simulink model "Main1"  (R2017b)
settings: Solver=ode15s  StartTime=0.0  StopTime=t_end  FixedStep=.0001  MaxStep=st  RelTol=1e-3  EnableMultiTasking=on
values from neighbouring files (symbols this model uses):
  A = eye(16,16)    [full_input_list.m]
  B = zeros(16,1)    [full_input_list.m]
  C = blkdiag(eye(3,3),zeros(3,3),eye(10,10))    [full_input_list.m]
  deltaT = 0.00001    (= 1e-05)    [full_input_list.m]
  H = C    [full_input_list.m]
  I_UD = [0.032808359, 0.000617048, 0.000049185;      0.000617048, 0.032531573, 0.000060042;      0.000049185, 0.000060042, 0.007799591]    [full_input_list.m]
  kd = 0.5    [full_input_list.m]    (also in initACS.m = 0.01)
  kd_UD_detumble = 6e-3    (= 0.006)    [full_input_list.m]
  kd_UD_slew = epsilon_UD_slew*.3    (= 0.003)    [full_input_list.m]
  kd_UD_spinUp = epsilon_UD_spinUp*0.025    (= 0.00025)    [full_input_list.m]
  kp = 1    [full_input_list.m]    (also in initACS.m = 0.01)
  kp_UD_slew = epsilon_UD_slew^2*.01    (= 1e-06)    [full_input_list.m]
  kp_UD_spinUp = epsilon_UD_spinUp^2*.05    (= 5e-06)    [full_input_list.m]
  magMomentMax_B = sat2CoilArea.*sat2n.*currentMax_B    [full_input_list.m]
  omega_cmd_N = 1e-1*[1 1 -.6]'    [full_input_list.m]
  omega_spinUp_MAG = 0.05    [full_input_list.m]
  OpModes = [0 0 0]    [full_input_list.m]
  OpTimes = [0 1 2]    [full_input_list.m]
  q4_cmd_init = [q4_cmd_init(2:4); q4_cmd_init(1)]    [full_input_list.m]
  Q_k = zeros(16,16)    [full_input_list.m]
  R = R_k    [full_input_list.m]
  sat2CoilArea = 0.8*[0.02; 0.02; 0.01]    [full_input_list.m]
  sat2n = [0; 100; 100]    [full_input_list.m]
  sat2Resistance = sat2WireLength.*sat2WireResistivity./sat2WireArea    [full_input_list.m]
  SeperationTime = 30000    [full_input_list.m]
  spinAxis_B = [1 0 0]    [full_input_list.m]
  st = 1/freq    (= 0.0125)    [full_input_list.m]    (also in initSimulink.m)
  u_k = zeros(16,1)    [full_input_list.m]
  w_k = zeros(16,1)    [full_input_list.m]
  Z_k = zeros(16,1)    [full_input_list.m]
undefined symbols (not defined in the file or in its folder): DiscIntNeverNeededParam, G_igrf, gyro_DCM_BS, H_igrf, I_B, IAU, Kschmidt, mag_variance, R_mean
libraries: aerolibutil x36, vrlib x31, SimMainLibrary x27, simulink x22, dspmathops x6, sharedtransform x4, sharedutil x2, dspinverses x2, dspmtrx3 x1, aerolibtransform2 x1, aerolibgravity2 x1, lib_violet_env x1
(part 2 of 3)

== system Main1/NEW/Flight Computers1/CenterCube EKF/Kalman Gain and Estamated State Computation ==
  P_kp : Inport
  x_kp : Inport  Port=2
  Y : Inport  Port=3
  " LU Inverse" : dspinverses/ LU Inverse
      settings: SourceProductName=DSP System Toolbox
  Add1 : Sum
  Add2 : Sum
  Add3 : Sum  Inputs=-+
  H : Constant  Value=H
  H1 : Constant  Value=H
  Math Function : Math  Operator=transpose  SaturateOnIntegerOverflow=on
  Product{,1,3..4,6} (5 alike) : Product  Multiplication=Matrix(*)
  Product2 : Product
  R : Constant  Value=R
  K : Outport
  x_k : Outport  Port=2
  wires:
  H/1 -> Product3/1, Product1/2, Math Function/1
  " LU Inverse"/1 -> Product/2
  Product1/1 -> Product/1
  Math Function/1 -> Product4/2
  Product/1 -> Product2/1, K/1  "Kalman Gain K"
  x_kp/1 -> Add2/1, Product6/2
  Y/1 -> Add3/2
  R/1 -> Add1/2
  Product4/1 -> Add1/1
  Add1/1 -> " LU Inverse"/1
  Product3/1 -> Product4/1
  H1/1 -> Product6/1
  Product6/1 -> Add3/1
  P_kp/1 -> Product3/2, Product1/1
  Add2/1 -> x_k/1
  Add3/1 -> Product2/2
  Product2/1 -> Add2/2

== system Main1/NEW/Flight Computers1/CenterCube EKF/New State Prediction  ==
  note: LKF
  note: EKF
  P_k-1 : Inport
  x_k-1 : Inport  Port=2
  A_LKF : Subsystem
  Add1 : Sum  Inputs=+++
  Add2 : Sum
  Add3 : Sum
  B : Constant  Value=B
  Math Function : Math  Operator=transpose  SaturateOnIntegerOverflow=on
  Math Function1 : Math  Operator=transpose  SaturateOnIntegerOverflow=on
  Predictions : Subsystem  TreatAsAtomicUnit=on
  Product{,1..5} (6 alike) : Product  Multiplication=Matrix(*)
  Q_k : Constant  Value=Q_k
  Q_k1 : Constant  Value=Q_k
  Terminator2 : Terminator
  Terminator3 : Terminator
  u_k : Constant  Value=u_k
  w_k : Constant  Value=w_k
  P_kp : Outport
  "x_kp  " : Outport  Port=2
  wires:
  Product2/1 -> Product3/1
  Math Function/1 -> Product3/2
  Product/1 -> Add1/1
  B/1 -> Product1/1
  Product1/1 -> Add1/2
  u_k/1 -> Product1/2
  w_k/1 -> Add1/3
  Q_k/1 -> Add2/2
  P_k-1/1 -> [A], Product2/2
  Product3/1 -> Add2/1
  x_k-1/1 -> Predictions/1(x_ko), Product/2, A_LKF/1(In1)
  A_LKF/1(Out1) -> Product2/1, Math Function/1, Product/1  "A"
  Predictions/1(F) -> Math Function1/1, Product4/1
  [A] -> Product4/2
  Product4/1 -> Product5/1
  Math Function1/1 -> Product5/2
  Predictions/2(x_kp) -> "x_kp  "/1  "x_kps"
  Product5/1 -> Add3/1
  Q_k1/1 -> Add3/2
  Add3/1 -> P_kp/1  "P_kp"
  Add2/1 -> Terminator2/1  "P_kp"
  Add1/1 -> Terminator3/1  "x_kp"

== system Main1/NEW/Flight Computers1/CenterCube EKF/Y computation ==
  In1 : Inport
  Add2 : Sum
  C : Constant  Value=C
  Product2 : Product  Multiplication=Matrix(*)
  "Z_k " : Constant  Value=Z_k
  Y : Outport
  wires:
  Add2/1 -> Y/1
  "Z_k "/1 -> Add2/2
  In1/1 -> Product2/2
  C/1 -> Product2/1
  Product2/1 -> Add2/1

== system Main1/NEW/Flight Computers1/CenterCube EKF/x_measured ==
  Sensor_data : Inport
  Bus Selector1 : BusSelector  OutputSignals=w_BN_1,magnetometer_1,sun_B,r_LLA,accelerometer_1,time
  Constant : Constant  Value=[0;0;0]
  Lookup Tables : Subsystem
  Terminator : Terminator
  Vector Concatenate : Concatenate  NumInputs=5
  q_N from Sensors : Subsystem
  x_measured : Outport
  B_N : Outport  Port=2
  wires:
  Bus Selector1/4 -> Vector Concatenate/1, Lookup Tables/1(x_pos)  "<r_LLA>"
  Vector Concatenate/1 -> x_measured/1
  Lookup Tables/2(V_sun_N) -> q_N from Sensors/4(V_sun_N)
  Bus Selector1/3 -> q_N from Sensors/2(V_sun_B)  "<sun_B>"
  Lookup Tables/1(B_N) -> B_N/1, q_N from Sensors/3(B_N)
  q_N from Sensors/2(Q) -> Terminator/1
  Sensor_data/1 -> Bus Selector1/1
  Bus Selector1/1 -> Vector Concatenate/4  "<w_BN_1>"
  Constant/1 -> Vector Concatenate/2  "xdot_measured"
  Bus Selector1/5 -> Vector Concatenate/3  "<accelerometer_1>"
  q_N from Sensors/1(q_N) -> Vector Concatenate/5  "quat_measured"
  Bus Selector1/2 -> q_N from Sensors/1(B_B)  "<magnetometer_1>"
  Bus Selector1/6 -> Lookup Tables/2(time)  "<time>"

== system Main1/NEW/Flight Computers1/Subsystem/Chart ==
  PwbMEX : Inport
  time : Inport  Port=2
  OpTimes : Inport  Port=3
  OpModes : Inport  Port=4
  SeparationTime : Inport  Port=5
  " Demux " : Demux  Outputs=1
  " SFunction " : S-Function  Tag=Stateflow S-Function Main 23  FunctionName=sf_sfun  PortCounts=[5 3]  SFunctionDeploymentMode=off  EnableBusSupport=on
  " Terminator " : Terminator
  OM : Outport
  SEPC : Outport  Port=2
  wires:
  PwbMEX/1 -> " SFunction "/1
  time/1 -> " SFunction "/2
  OpTimes/1 -> " SFunction "/3
  OpModes/1 -> " SFunction "/4
  SeparationTime/1 -> " SFunction "/5
  " SFunction "/2 -> OM/1  "OM"
  " SFunction "/3 -> SEPC/1  "SEPC"
  " Demux "/1 -> " Terminator "/1
  " SFunction "/1 -> " Demux "/1

== system Main1/NEW/Sensors1/Center Cube Sensors/Create Mag Vector ==
  q_BN : Inport
  r_N : Inport  Port=2
  Constant : Constant  Value=[1 1 1]
  Terminator : Terminator
  Terminator1 : Terminator
  mag_B : Outport
  wires:
  Constant/1 -> mag_B/1
  r_N/1 -> Terminator1/1
  q_BN/1 -> Terminator/1

== system Main1/NEW/Sensors1/Center Cube Sensors/Create Sun Vector ==
  note: s_hat_N
  note: Outputs the unit vector towards the sun wrt the body (or earth; doesn't matter) in the inertial frame (N).
  q_BN : Inport
  GPS time : Inport  Port=2
  GPS time to Jd sfrom J2000 : Subsystem
  Normalization : dspmathops/Normalization  NormType=2-norm  Bias=1e-10  NormOver=Each column  Dimension=1  outputDataTypeStr=Inherit: Same as product output  outputLastDataTypeStr=Inherit: Same as product output  outputMin=[]  outputMax=[]  accumDataTypeStr=Inherit: Same as product output  accumLastDataTypeStr=Inherit: Same as product output  roundingMode=Floor  overflowMode=off
      settings: SourceProductName=DSP System Toolbox
  Product : Product  Multiplication=Matrix(*)
  Quaternions to Direction Cosine Matrix : sharedtransform/Quaternions to  Direction Cosine Matrix
      settings: SourceProductName=Aerospace Blockset  SourceProductBaseCode=AE
  Sun position off of Jd frm J2000 : Subsystem
  sun_B : Outport
  wires:
  GPS time/1 -> GPS time to Jd sfrom J2000/1(In1)
  Product/1 -> sun_B/1
  q_BN/1 -> Quaternions to Direction Cosine Matrix/1
  Normalization/1 -> Product/2
  Quaternions to Direction Cosine Matrix/1 -> Product/1
  GPS time to Jd sfrom J2000/1(Out1) -> Sun position off of Jd frm J2000/1(In1)
  Sun position off of Jd frm J2000/1(Out1) -> Normalization/1

== system Main1/NEW/Sensors1/Center Cube Sensors/GPS ==
  note: Position in the sensor reference frame
  note: GPS Sensor Spoofing
      | We must specify the GPS variance and seed later when we have more time
      |
      | DCM of ECFE wrt ECI is not filled in
      |
      | GPS start time needs to be filled in.
      |
      | Violet was able to check for corrupt signals - that is the next step
  note: Velocity in the sensor reference frame
  r_N : Inport
  v_N : Inport  Port=2
  DCM of ECFC wrt ECI : Constant  Value=eye(3)
  DCM of ECFC wrt ECI1 : Constant  Value=eye(3)
  Digital Clock : DigitalClock
  GPS start time : Constant  Value=0
  Position random noise : RandomNumber  SampleTime=0.1
  Product : Product
  Product1 : Product
  Sum : Sum
  Sum1 : Sum
  Sum2 : Sum  Inputs=|++
  Velocity random noise : RandomNumber  SampleTime=0.1
  r_S : Outport
  v_S : Outport  Port=2
  Time : Outport  Port=3
  wires:
  Sum/1 -> r_S/1
  Position random noise/1 -> Sum/2
  Sum1/1 -> v_S/1
  Velocity random noise/1 -> Sum1/2
  GPS start time/1 -> Sum2/1
  Digital Clock/1 -> Sum2/2
  Sum2/1 -> Time/1
  DCM of ECFC wrt ECI/1 -> Product/1
  r_N/1 -> Product/2
  Product/1 -> Sum/1
  DCM of ECFC wrt ECI1/1 -> Product1/1
  v_N/1 -> Product1/2
  Product1/1 -> Sum1/1

== system Main1/NEW/Sensors1/Center Cube Sensors/Gyro ==
  note: Gyro Sensor Spoofing
      |
      | Lots of work left to be done on the Gyro. Violet tracks the gyro bias - necessary?
      |
      | Violet also records the time of the gyro - is this simply a diagnostic step?
  w_BN_B : Inport
  Bias : Subsystem  TreatAsAtomicUnit=on
  Bus Creator : BusCreator  Inputs=2
  Digital Clock : DigitalClock
  Discrete-Time Integrator : DiscreteIntegrator  gainval=1  InitialConditionSetting=State (most efficient)  ICPrevOutput=DiscIntNeverNeededParam  ICPrevScaledInput=DiscIntNeverNeededParam
  Gyro_DCM_BS : Constant  Value=gyro_DCM_BS
  Product : Product  Multiplication=Matrix(*)
  Random Bias Steps : RandomNumber  SampleTime=0.1
  Random Noise : RandomNumber  SampleTime=0.1
  Sum : Sum
  w_SN_S_m : Outport
  time : Outport  Port=2
  Gyro : Outport  Port=3
  wires:
  w_BN_B/1 -> Product/2
  Random Bias Steps/1 -> Discrete-Time Integrator/1
  Product/1 -> Sum/1
  Discrete-Time Integrator/1 -> Sum/2
  Sum/1 -> Bias/1(w)
  Random Noise/1 -> Bias/2(noise)
  Bias/1(wn) -> Bus Creator/1, w_SN_S_m/1
  Gyro_DCM_BS/1 -> Product/1
  Digital Clock/1 -> Bus Creator/2, time/1
  Bus Creator/1 -> Gyro/1

== system Main1/NEW/Sensors1/Center Cube Sensors/Magnetometer ==
  note: Teslas to Gauss
  note: from r_E to b_B is in Violet Dynamics Block.
      | The rest is in their sensor block.
  note: b_B
  note: DCM of Body wrt Neutral
  note: Pulled from NASA Langley
  note: The block takes the magnetic field in the body reference frame
      | and transforms it into magnetic field in the sensor reference
      | frame.
      |
      | We still need the DCM and the variance of the magnetometer
  r_E : Inport  PortDimensions=[1 3]
  Bus Creator : BusCreator  Inputs=2
  DCM B wrt S : Constant  Value=eye(3)
  DCM of BN : Constant  Value=eye(3)
  DCM of ECFC wrt ECI : Constant  Value=eye(3)
  Digital Clock : DigitalClock
  Gain : Gain  Gain=1e4
  Magnetic Field Model : Subsystem
  Math Function : Math  Operator=transpose  SaturateOnIntegerOverflow=on
  Math Function1 : Math  Operator=transpose  SaturateOnIntegerOverflow=on
  Matrix Multiply : Product  Multiplication=Matrix(*)
  Matrix Multiply1 : Product  Multiplication=Matrix(*)
  Product : Product  Multiplication=Matrix(*)
  Random Number : RandomNumber  Variance=mag_variance  SampleTime=0.1
  Sine Wave : Sin  Amplitude=0 * 1e-6 * randn(3, 1)  Frequency=2*pi / (90 * 60)  SampleTime=0
  Sum : Sum  Inputs=|++
  Sum1 : Sum  Inputs=|++
  b_S : Outport
  Time : Outport  Port=2
  Magnetometer : Outport  Port=3
  wires:
  Matrix Multiply1/1 -> Sum/1
  Random Number/1 -> Sum/2
  DCM B wrt S/1 -> Math Function/1
  Sum/1 -> Product/2
  Math Function/1 -> Product/1
  Product/1 -> Gain/1
  Gain/1 -> Bus Creator/1, b_S/1
  r_E/1 -> Magnetic Field Model/1(r_E)
  Magnetic Field Model/1(b_E) -> Sum1/1
  Sine Wave/1 -> Sum1/2
  Sum1/1 -> Matrix Multiply/2
  Math Function1/1 -> Matrix Multiply/1
  Matrix Multiply/1 -> Matrix Multiply1/2
  DCM of ECFC wrt ECI/1 -> Math Function1/1
  DCM of BN/1 -> Matrix Multiply1/1
  Digital Clock/1 -> Bus Creator/2, Time/1
  Bus Creator/1 -> Magnetometer/1

== system Main1/NEW/Sensors1/Center Cube Sensors/Sun Sensor ==
  In1 : Inport
  Out1 : Outport
  wires:
  In1/1 -> Out1/1

== system Main1/NEW/Flight Computers1/Center Cube Controller/Attitude Compensator/Chart ==
  q : Inport
  qCmd : Inport  Port=2
  etaB : Inport  Port=3
  BN : Inport  Port=4
  w_BN_N : Inport  Port=5
  w_errN : Inport  Port=6
  KpSU : Inport  Port=7
  KdSU : Inport  Port=8
  I_B : Inport  Port=9
  SafeSEPC : Inport  Port=10
  SafeOM : Inport  Port=11
  KpS : Inport  Port=12
  KdS : Inport  Port=13
  " Demux " : Demux
  " SFunction " : S-Function  Tag=Stateflow S-Function Main 14  FunctionName=sf_sfun  PortCounts=[21 25]  SFunctionDeploymentMode=off  EnableBusSupport=on
  TorqueD : Subsystem
      settings: UndoDeleteFcn=Stateflow.SLINSF.SimulinkMan.restorePreDeleteFcn  PreDeleteFcn=Stateflow.SLINSF.SimulinkMan.removePreDeleteFcn
  TorqueDeployed : Subsystem
      settings: UndoDeleteFcn=Stateflow.SLINSF.SimulinkMan.restorePreDeleteFcn  PreDeleteFcn=Stateflow.SLINSF.SimulinkMan.removePreDeleteFcn
  TorquePD_Slew : Subsystem
      settings: UndoDeleteFcn=Stateflow.SLINSF.SimulinkMan.restorePreDeleteFcn  PreDeleteFcn=Stateflow.SLINSF.SimulinkMan.removePreDeleteFcn
  TorquePD_SpinUp : Subsystem
      settings: UndoDeleteFcn=Stateflow.SLINSF.SimulinkMan.restorePreDeleteFcn  PreDeleteFcn=Stateflow.SLINSF.SimulinkMan.removePreDeleteFcn
  P : Outport
  D : Outport  Port=2
  T_N : Outport  Port=3
  wires:
  q/1 -> " SFunction "/1
  qCmd/1 -> " SFunction "/2
  etaB/1 -> " SFunction "/3
  BN/1 -> " SFunction "/4
  w_BN_N/1 -> " SFunction "/5
  w_errN/1 -> " SFunction "/6
  KpSU/1 -> " SFunction "/7
  KdSU/1 -> " SFunction "/8
  I_B/1 -> " SFunction "/9
  SafeSEPC/1 -> " SFunction "/10
  SafeOM/1 -> " SFunction "/11
  KpS/1 -> " SFunction "/12
  KdS/1 -> " SFunction "/13
  " SFunction "/2 -> P/1  "P"
  " SFunction "/3 -> D/1  "D"
  " SFunction "/4 -> T_N/1  "T_N"
  " SFunction "/5 -> TorquePD_Slew/1(q)
  " SFunction "/6 -> TorquePD_Slew/2(qCmd)
  " SFunction "/7 -> TorquePD_Slew/3(etaB)
  " SFunction "/8 -> TorquePD_Slew/4(BN)
  " SFunction "/9 -> TorquePD_Slew/5(w_errN)
  " SFunction "/10 -> TorquePD_Slew/6(KpS)
  " SFunction "/11 -> TorquePD_Slew/7(KdS)
  " SFunction "/12 -> TorquePD_Slew/8(I_B)
  TorquePD_Slew/1(P) -> " SFunction "/14
  TorquePD_Slew/2(D) -> " SFunction "/15
  TorquePD_Slew/3(T_N) -> " SFunction "/16
  " Demux "/1 -> TorquePD_Slew/Trigger
  " SFunction "/13 -> TorqueD/1(w_BN_N)
  " SFunction "/14 -> TorqueD/2(I_B)
  " SFunction "/15 -> TorqueD/3(q)
  TorqueD/1(T_N) -> " SFunction "/17
  " Demux "/2 -> TorqueD/Trigger
  " SFunction "/16 -> TorqueDeployed/1(q)
  " SFunction "/17 -> TorqueDeployed/2(w_BN_N)
  TorqueDeployed/1(T_N) -> " SFunction "/18
  " Demux "/3 -> TorqueDeployed/Trigger
  " SFunction "/18 -> TorquePD_SpinUp/1(q)
  " SFunction "/19 -> TorquePD_SpinUp/2(qCmd)
  " SFunction "/20 -> TorquePD_SpinUp/3(etaB)
  " SFunction "/21 -> TorquePD_SpinUp/4(BN)
  " SFunction "/22 -> TorquePD_SpinUp/5(w_errN)
  " SFunction "/23 -> TorquePD_SpinUp/6(KpSU)
  " SFunction "/24 -> TorquePD_SpinUp/7(KdSU)
  " SFunction "/25 -> TorquePD_SpinUp/8(I_B)
  TorquePD_SpinUp/1(P) -> " SFunction "/19
  TorquePD_SpinUp/2(D) -> " SFunction "/20
  TorquePD_SpinUp/3(T_N) -> " SFunction "/21
  " Demux "/4 -> TorquePD_SpinUp/Trigger
  " SFunction "/1 -> " Demux "/1

== system Main1/NEW/Flight Computers1/Center Cube Controller/Attitude Compensator/Commanded state ==
  Bus Creator : BusCreator  Inputs=2
  Quaternion Integration : Subsystem
  omega_N : Constant  Value=omega_cmd_N
  q : Constant  Commented=on  Value=[0 0 0 1]'
  State_cmd : Outport
  wires:
  Quaternion Integration/1(q4) -> Bus Creator/1  "q4_cmd"
  omega_N/1 -> Bus Creator/2, Quaternion Integration/1(w_N)  "omega_cmd_N"
  Bus Creator/1 -> State_cmd/1

== system Main1/NEW/Flight Computers1/Center Cube Controller/Attitude Compensator/Deployed Modes (switch)1 ==
  note: Deployed Block
      | Notes: This block determines the actions the satellite will execute based on the commands given by ground control/ powerboard. The 2 cases are normal operations, and eclipse
  Mode and BurnCmd : Inport
  Attitude State : Inport  Port=2
  Action Port : ActionPort  ActionType=case
  Bus Selector : BusSelector  OutputSignals=SafedOpMode,SeperationCommand
  Bus Selector1 : BusSelector  OutputSignals=q_BN_est,w_BN_est
  Default : Subsystem  TreatAsAtomicUnit=on
  Deployed : SwitchCase  CaseConditions={7, 12}
  Merge1 : Merge  Inputs=3
  Seek EKF Convergence : Subsystem  TreatAsAtomicUnit=on
  Spin-Up Slew : Subsystem  TreatAsAtomicUnit=on
  Terminator : Terminator
  Out1 : Outport
  wires:
  Deployed/1 -> Spin-Up Slew/Action
  Spin-Up Slew/1(tau) -> Merge1/1
  Attitude State/1 -> Bus Selector1/1
  Deployed/3 -> Default/Action
  Merge1/1 -> Out1/1
  Mode and BurnCmd/1 -> Bus Selector/1
  Bus Selector/1 -> Deployed/1  "<SafedOpMode>"
  Bus Selector/2 -> Terminator/1  "<SeperationCommand>"
  Default/1(Out1) -> Merge1/3
  Deployed/2 -> Seek EKF Convergence/Action
  Seek EKF Convergence/1(Out1) -> Merge1/2
  Bus Selector1/1 -> Spin-Up Slew/1(q)  "<q_BN_est>"
  Bus Selector1/2 -> Spin-Up Slew/2(w)  "<w_BN_est>"

== system Main1/NEW/Flight Computers1/Center Cube Controller/Attitude Compensator/Not Deployed Modes (switch) ==
  note: What is the seek EKF Convergence?
  note: Not Deployed Block
      | Notes: This block determines the actions the satellite will execute based on the commands given by ground control/ powerboard. The 3 cases are detumbling, sun pointing, and eclipse
  Mode and BurnCmd : Inport
  q_BN : Inport  Port=2
  w_BN : Inport  Port=3
  Action Port : ActionPort
  Bus Selector : BusSelector  OutputSignals=SafedOpMode,SeperationCommand
  Detumbling Slew : Subsystem  TreatAsAtomicUnit=on
  Inertia : Constant  Value=I_UD
  Inital Spin Up : Subsystem  TreatAsAtomicUnit=on
  Merge1 : Merge  Inputs=5
  Not Deployed : SwitchCase  CaseConditions={5,6,7,12}
  Null Case1 : Subsystem  TreatAsAtomicUnit=on
  Seek EKF Convergence : Subsystem  TreatAsAtomicUnit=on
  Sun Pointing : Subsystem  TreatAsAtomicUnit=on
  Terminator : Terminator
  Out1 : Outport
  wires:
  Merge1/1 -> Out1/1
  Not Deployed/5 -> Null Case1/Action
  q_BN/1 -> Sun Pointing/1(q), Inital Spin Up/1(q_BN), Detumbling Slew/1(q_BN)
  Detumbling Slew/1(tau) -> Merge1/1
  Not Deployed/2 -> Sun Pointing/Action
  Sun Pointing/1(tau) -> Merge1/2
  Not Deployed/1 -> Detumbling Slew/Action
  w_BN/1 -> Detumbling Slew/2(w_BN), Sun Pointing/2(w_BN), Inital Spin Up/2(w)
  Mode and BurnCmd/1 -> Bus Selector/1
  Not Deployed/3 -> Inital Spin Up/Action
  Inital Spin Up/1(tau) -> Merge1/3
  Inertia/1 -> Inital Spin Up/3("I "), Detumbling Slew/3("Inertia ")
  Not Deployed/4 -> Seek EKF Convergence/Action
  Null Case1/1(Out1) -> Merge1/5
  Seek EKF Convergence/1(Out1) -> Merge1/4
  Bus Selector/1 -> Not Deployed/1  "<SafedOpMode>"
  Bus Selector/2 -> Terminator/1  "<SeperationCommand>"

== system Main1/NEW/Flight Computers1/Center Cube Controller/Attitude Compensator/Subsystem ==
  v : Inport
  Constant : Constant  Value=[0;0;0]
  Dot Product : DotProduct  InputSameDT=on  OutDataTypeStr=Inherit: Inherit via internal rule
  Sqrt : Sqrt  SaturateOnIntegerOverflow=on
  Sum of Elements : Sum  Inputs=+
  Switch : Switch  Criteria=u2 ~= 0
  multiply : Product  Inputs=*/
  v_hat : Outport
  wires:
  v/1 -> Dot Product/2, Dot Product/1, multiply/1
  Switch/1 -> v_hat/1
  Constant/1 -> Switch/3
  multiply/1 -> Switch/1
  Sum of Elements/1 -> Sqrt/1
  Dot Product/1 -> Sum of Elements/1
  Sqrt/1 -> Switch/2, multiply/2

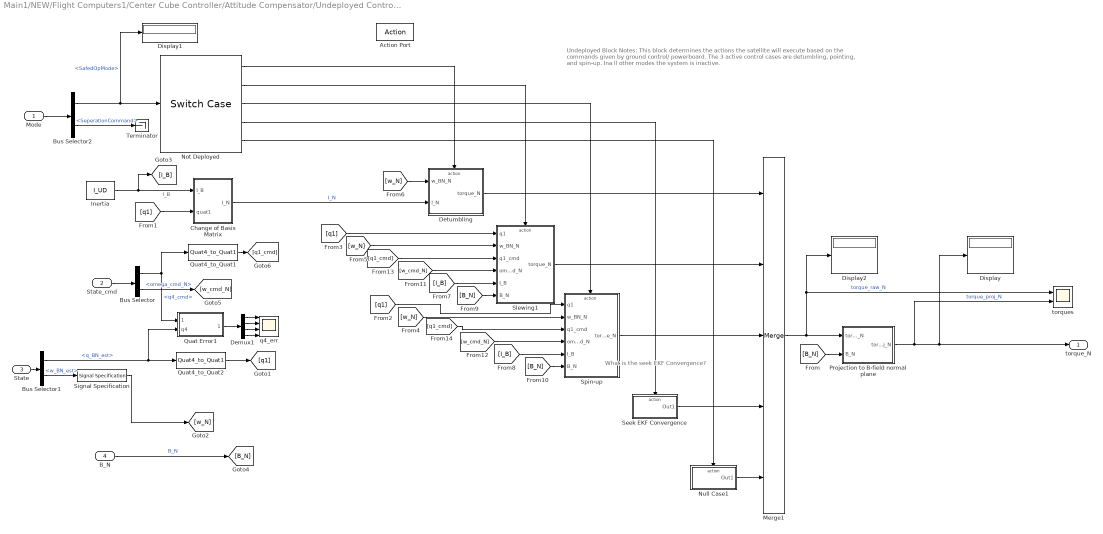
== system Main1/NEW/Flight Computers1/Center Cube Controller/Attitude Compensator/Undeployed Control Modes ==
  note: What is the seek EKF Convergence?
  note: Undeployed Block
      | Notes: This block determines the actions the satellite will execute based on the commands given by ground control/ powerboard. The 3 active control cases are detumbling, pointing, and spin-up. Ina ll other modes the system is inactive.
  Mode : Inport
  State_cmd : Inport  Port=2
  State : Inport  Port=3
  B_N : Inport  Port=4
  Action Port : ActionPort  ActionType=case
  Bus Selector : BusSelector  OutputSignals=q4_cmd,omega_cmd_N
  Bus Selector1 : BusSelector  OutputSignals=q_BN_est,w_BN_est
  Bus Selector2 : BusSelector  OutputSignals=SafedOpMode,SeperationCommand
  Change of Basis Matrix : Subsystem
  Demux1 : Demux
  Detumbling : Subsystem  TreatAsAtomicUnit=on
  Display : Display
  Display1 : Display
  Display2 : Display
  Inertia : Constant  Value=I_UD
  Merge1 : Merge  Inputs=5
  Not Deployed : SwitchCase  CaseConditions={5,6,7,12}
  Null Case1 : Subsystem  TreatAsAtomicUnit=on
  Projection to B-field normal plane : Subsystem
  Quat Error1 : Subsystem
  Quat4_to_Quat1 : SimMainLibrary/Quat4_to_Quat1
      settings: SourceProductName=CUGravity Library
  Quat4_to_Quat2 : SimMainLibrary/Quat4_to_Quat1
      settings: SourceProductName=CUGravity Library
  Seek EKF Convergence : Subsystem  TreatAsAtomicUnit=on
  Signal Specification : SignalSpecification  OutDataTypeStr=double  Dimensions=3
  Slewing1 : Subsystem  TreatAsAtomicUnit=on
  Spin-up : Subsystem  TreatAsAtomicUnit=on
  Terminator : Terminator
  q4_err : Scope  NumInputPorts=4
  torques : Scope  NumInputPorts=2
  torque_N : Outport
  wires:
  Merge1/1 -> Display2/1, torques/1, Projection to B-field normal plane/1(torque_raw_N)  "torque_raw_N"
  Not Deployed/5 -> Null Case1/Action
  Bus Selector1/1 -> Quat Error1/2(q4), Quat4_to_Quat2/1  "<q_BN_est>"
  Detumbling/1(torque_N) -> Merge1/1
  Not Deployed/2 -> Slewing1/Action
  Not Deployed/1 -> Detumbling/Action
  Bus Selector1/2 -> Signal Specification/1  "<w_BN_est>"
  Not Deployed/3 -> Spin-up/Action
  Spin-up/1(torque_N) -> Merge1/3
  Inertia/1 -> Change of Basis Matrix/1(I_B), [I_B]  "I_B"
  Not Deployed/4 -> Seek EKF Convergence/Action
  Null Case1/1(Out1) -> Merge1/5
  Seek EKF Convergence/1(Out1) -> Merge1/4
  State_cmd/1 -> Bus Selector/1
  State/1 -> Bus Selector1/1
  Bus Selector/1 -> Quat4_to_Quat1/1, Quat Error1/1(q4_command)  "<q4_cmd>"
  Quat4_to_Quat1/1 -> [q1_cmd]
  Change of Basis Matrix/1(I_N) -> Detumbling/2(I_N)  "I_N"
  B_N/1 -> [B_N]  "B_N"
  Projection to B-field normal plane/1(torque_proj_N) -> torques/2, torque_N/1, Display/1  "torque_proj_N"
  Quat4_to_Quat2/1 -> [q1]
  Slewing1/1(torque_N) -> Merge1/2
  Demux1/2 -> q4_err/2
  Demux1/3 -> q4_err/3
  Demux1/1 -> q4_err/1
  Demux1/4 -> q4_err/4
  Quat Error1/1(q4_error) -> Demux1/1
  Bus Selector/2 -> [w_cmd_N]  "<omega_cmd_N>"
  [q1] -> Change of Basis Matrix/2(quat1)
  [q1] -> Spin-up/1(q1)
  [q1] -> Slewing1/1(q1)
  [w_N] -> Spin-up/2(w_BN_N)
  [w_N] -> Slewing1/2(w_BN_N)
  [w_N] -> Detumbling/1(w_BN_N)
  [I_B] -> Slewing1/5(I_B)
  [I_B] -> Spin-up/5(I_B)
  [B_N] -> Slewing1/6(B_N)
  [B_N] -> Spin-up/6(B_N)
  [w_cmd_N] -> Slewing1/4(omegaCmd_N)
  [w_cmd_N] -> Spin-up/4(omegaCmd_N)
  [q1_cmd] -> Slewing1/3(q1_cmd)
  [q1_cmd] -> Spin-up/3(q1_cmd)
  Bus Selector2/2 -> Terminator/1  "<SeperationCommand>"
  Bus Selector2/1 -> Display1/1, Not Deployed/1  "<SafedOpMode>"
  Mode/1 -> Bus Selector2/1
  Signal Specification/1 -> [w_N]
  [B_N] -> Projection to B-field normal plane/2(B_N)

== system Main1/NEW/Flight Computers1/Center Cube Controller/Motor Control Placeholder/Spinning fast ==
  Action Port : ActionPort
  Constant : Constant  Value=0.05
  Out1 : Outport
  wires:
  Constant/1 -> Out1/1

== system Main1/NEW/Flight Computers1/Center Cube Controller/Motor Control Placeholder/Spinning slow ==
  Action Port : ActionPort
  Constant : Constant  Value=0
  Out1 : Outport
  wires:
  Constant/1 -> Out1/1

== system Main1/NEW/Flight Computers1/Center Cube Controller/SafeMode/Chart1 ==
  PbOpMode : Inport
  Mag1 : Inport  Port=2
  Mag2 : Inport  Port=3
  Acc1 : Inport  Port=4
  Acc2 : Inport  Port=5
  Gyro1 : Inport  Port=6
  Gyro2 : Inport  Port=7
  Sun1 : Inport  Port=8
  Sun2 : Inport  Port=9
  MagX1 : Inport  Port=10
  MagY1 : Inport  Port=11
  MagZ1 : Inport  Port=12
  EKFAE : Inport  Port=13
  EKFhs : Inport  Port=14
  SafeMode_In : Inport  Port=15
  t : Inport  Port=16
  OpMode : Inport  Port=17
  SeperationCommand : Inport  Port=18
  " Demux " : Demux  Outputs=1
  " SFunction " : S-Function  Tag=Stateflow S-Function Main 24  FunctionName=sf_sfun  PortCounts=[18 4]  SFunctionDeploymentMode=off  EnableBusSupport=on
  " Terminator " : Terminator
  OpMode_Out : Outport
  PwbMEX : Outport  Port=2
  SafeMode_Out : Outport  Port=3
  wires:
  PbOpMode/1 -> " SFunction "/1
  Mag1/1 -> " SFunction "/2
  Mag2/1 -> " SFunction "/3
  Acc1/1 -> " SFunction "/4
  Acc2/1 -> " SFunction "/5
  Gyro1/1 -> " SFunction "/6
  Gyro2/1 -> " SFunction "/7
  Sun1/1 -> " SFunction "/8
  Sun2/1 -> " SFunction "/9
  MagX1/1 -> " SFunction "/10
  MagY1/1 -> " SFunction "/11
  MagZ1/1 -> " SFunction "/12
  EKFAE/1 -> " SFunction "/13
  EKFhs/1 -> " SFunction "/14
  SafeMode_In/1 -> " SFunction "/15
  t/1 -> " SFunction "/16
  OpMode/1 -> " SFunction "/17
  SeperationCommand/1 -> " SFunction "/18
  " SFunction "/2 -> OpMode_Out/1  "OpMode_Out"
  " SFunction "/3 -> PwbMEX/1  "PwbMEX"
  " SFunction "/4 -> SafeMode_Out/1  "SafeMode_Out"
  " Demux "/1 -> " Terminator "/1
  " SFunction "/1 -> " Demux "/1

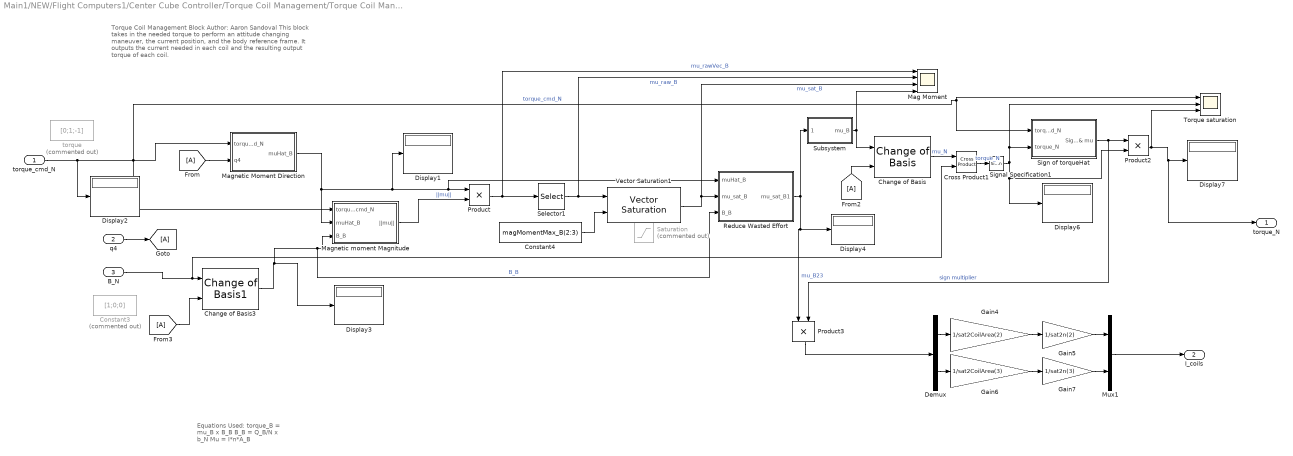
== system Main1/NEW/Flight Computers1/Center Cube Controller/Torque Coil Management/Torque Coil Management ==
  note: Equations Used:
      |
      | torque_B = mu_B x B_B
      |
      | B_B = Q_B/N x b_N
      |
      | Mu = I*n*A_B
  note: Torque Coil Management Block
      | Author: Aaron Sandoval
      | This block takes in the needed torque to perform an attitude
      | changing maneuver, the current position, and the body reference
      | frame. It outputs the current needed in each coil and the resulting
      | output torque of each coil.
  torque_cmd_N : Inport
  q4 : Inport  Port=2
  B_N : Inport  Port=3
  Change of Basis : SimMainLibrary/Change of Basis
      settings: SourceProductName=CUGravity Library
  Change of Basis3 : SimMainLibrary/Change of Basis1
      settings: SourceProductName=CUGravity Library
  Constant3 : Constant  Commented=on  Value=[1;0;0]
  Constant4 : Constant  Value=magMomentMax_B(2:3)
  Cross Product1 : vrlib/Utilities/Cross Product
      settings: SourceProductBaseCode=VR
  Demux : Demux  Outputs=2
  Display{1..4,6..7} (6 alike) : Display
  Gain4 : Gain  Gain=1/sat2CoilArea(2)
  Gain5 : Gain  Gain=1/sat2n(2)
  Gain6 : Gain  Gain=1/sat2CoilArea(3)
  Gain7 : Gain  Gain=1/sat2n(3)
  Mag Moment : Scope  NumInputPorts=4
  Magnetic Moment Direction : Subsystem
  Magnetic moment Magnitude : Subsystem
  Mux1 : Mux  Inputs=2
  Product : Product
  Product2 : Product
  Product3 : Product
  Reduce Wasted Effort : Subsystem
  Saturation : Saturate  Commented=on  UpperLimit=magMomentMax_B(2:3)  LowerLimit=-magMomentMax_B(2:3)
  Selector1 : Selector  InputPortWidth=3  IndexOptions=Index vector (dialog)  Indices=[2 3]  OutputSizes=1
  Sign of torqueHat : Subsystem
  Signal Specification1 : SignalSpecification  OutDataTypeStr=double  Dimensions=3
  Subsystem : Subsystem
  Torque saturation : Scope  NumInputPorts=3
  Vector Saturation1 : SimMainLibrary/Vector Saturation
      settings: SourceProductName=CUGravity Library
  torque : Constant  Commented=on  Value=[0;1;-1]
  torque_N : Outport
  I_coils : Outport  Port=2
  wires:
  q4/1 -> [A]
  Change of Basis/1 -> Cross Product1/1  "mu_N"
  torque_cmd_N/1 -> Display2/1, Sign of torqueHat/1(torque_cmd_N), Torque saturation/1, Magnetic Moment Direction/1(torque_cmd_N), Magnetic moment Magnitude/1(torque_cmd_N)  "torque_cmd_N"
  Mux1/1 -> I_coils/1
  [A] -> Change of Basis/2
  Selector1/1 -> Vector Saturation1/1, Mag Moment/2  "mu_raw_B"
  Cross Product1/1 -> Signal Specification1/1  "torque_N"
  Gain4/1 -> Gain5/1
  Change of Basis3/1 -> Display3/1, Reduce Wasted Effort/3(B_B), Magnetic moment Magnitude/3(B_B)  "B_B"
  Product/1 -> Mag Moment/1, Selector1/1  "mu_rawVec_B"
  Magnetic moment Magnitude/1(||mu||) -> Product/2  "||mu||"
  Gain6/1 -> Gain7/1
  Demux/2 -> Gain6/1
  Demux/1 -> Gain4/1
  Gain7/1 -> Mux1/2
  Gain5/1 -> Mux1/1
  B_N/1 -> Cross Product1/2, Change of Basis3/1
  [A] -> Change of Basis3/2
  Reduce Wasted Effort/1(mu_sat_B1) -> Product3/1, Display4/1, Subsystem/1(mu_B23)  "mu_B23"
  Vector Saturation1/1 -> Reduce Wasted Effort/2(mu_sat_B), Mag Moment/3  "mu_sat_B"
  Constant4/1 -> Vector Saturation1/2
  Product2/1 -> Torque saturation/3, torque_N/1, Display7/1
  Product3/1 -> Demux/1
  Sign of torqueHat/1(Sign_B & mu) -> Product3/2, Product2/1  "sign multiplier"
  Magnetic Moment Direction/1(muHat_B) -> Magnetic moment Magnitude/2(muHat_B), Reduce Wasted Effort/1(muHat_B), Product/1, Display1/1
  [A] -> Magnetic Moment Direction/2(q4)
  Subsystem/1(mu_B) -> Change of Basis/1, Mag Moment/4
  Signal Specification1/1 -> Product2/2, Display6/1, Sign of torqueHat/2(torque_N), Torque saturation/2

== system Main1/NEW/Flight Computers1/CenterCube EKF/New State Prediction /A_LKF ==
  In1 : Inport
  A : Constant  Value=A
  A1 : Constant  Value=deltaT/2
  A2 : Constant  Value=[0 0 0 1; 0 0 1 0; 0 -1 0 0; -1 0 0 0];
  A3 : Constant  Value=[0 0 -1 0; 0 0 0 1; 1 0 0 0; 0 1 0 0];
  A4 : Constant  Value=[0 1 0 0;-1 0 0 0; 0 0 0 1; 0 0 -1 0];
  Demux : Demux  Outputs=16
  MATLAB Function : Subsystem  TreatAsAtomicUnit=on
  Matrix Concatenate : Concatenate  NumInputs=3  Mode=Multidimensional array  ConcatenateDimension=2
  Mux : Mux
  Product4 : Product  Multiplication=Matrix(*)
  Product5 : Product  Multiplication=Matrix(*)
  Product6 : Product  Multiplication=Matrix(*)
  Product7 : Product
  Terminator{,1..11} (12 alike) : Terminator
  Out1 : Outport
  wires:
  In1/1 -> Demux/1
  Demux/4 -> Terminator3/1
  Demux/5 -> Terminator4/1
  Demux/3 -> Terminator2/1
  Demux/6 -> Terminator5/1
  Demux/9 -> Terminator8/1
  Demux/10 -> Terminator9/1
  Demux/7 -> Terminator6/1
  Demux/8 -> Terminator7/1
  Demux/12 -> Terminator11/1
  Demux/11 -> Terminator10/1
  Demux/13 -> Mux/1
  Demux/16 -> Mux/4
  Demux/15 -> Mux/3
  Demux/14 -> Mux/2
  Demux/1 -> Terminator/1
  Mux/1 -> Product4/2, Product6/2, Product5/2
  Product4/1 -> Matrix Concatenate/1
  A3/1 -> Product5/1
  Product6/1 -> Matrix Concatenate/3
  A4/1 -> Product6/1
  Matrix Concatenate/1 -> Product7/2
  A2/1 -> Product4/1
  Product7/1 -> MATLAB Function/2(replacement)
  MATLAB Function/1(A) -> Out1/1
  A1/1 -> Product7/1
  Product5/1 -> Matrix Concatenate/2
  Demux/2 -> Terminator1/1
  A/1 -> MATLAB Function/1("A ")

== system Main1/NEW/Flight Computers1/CenterCube EKF/New State Prediction /Predictions ==
  x_ko : Inport
  " Demux " : Demux  Outputs=1
  " SFunction " : S-Function  Tag=Stateflow S-Function Main 16  FunctionName=sf_sfun  PortCounts=[1 3]  SFunctionDeploymentMode=off  EnableBusSupport=on
  " Terminator " : Terminator
  F : Outport
  x_kp : Outport  Port=2
  wires:
  x_ko/1 -> " SFunction "/1
  " SFunction "/2 -> F/1  "F"
  " SFunction "/3 -> x_kp/1  "x_kp"
  " Demux "/1 -> " Terminator "/1
  " SFunction "/1 -> " Demux "/1

== system Main1/NEW/Flight Computers1/CenterCube EKF/x_measured/Lookup Tables ==
  note: r_N is in format:
      | - Lat (N-S) in decimal deg
      | - Long (E-W) in decimal deg
      | - Height in m
  x_pos : Inport
  time : Inport  Port=2
  Demux : Demux  Outputs=3
  ECI Position to LLA : aerolibtransform2/ECI Position to LLA  Commented=on  red=IAU-2000/2006  year=2016  month=September  day=20  hour=0  min=0  sec=0  deltaT=Sec  errorflag=Error  extraparamflag=off  eunits=Metric (MKS)  earthmodel=WGS84  flat=1/298.257223563  eqradius=6378137
      settings: AttributesFormatString=%<red>  SourceProductName=Aerospace Blockset  SourceProductBaseCode=AE
  GPS time to Jd sfrom J2000 : Subsystem
  Normalization : dspmathops/Normalization  NormType=2-norm  Bias=1e-10  NormOver=Each column  Dimension=1  outputDataTypeStr=Inherit: Same as product output  outputLastDataTypeStr=Inherit: Same as product output  outputMin=[]  outputMax=[]  accumDataTypeStr=Inherit: Same as product output  accumLastDataTypeStr=Inherit: Same as product output  roundingMode=Floor  overflowMode=off
      settings: SourceProductName=DSP System Toolbox
  "RBF!!!!! " : Constant  Value=2015
  Sun position off of Jd frm J2000 : Subsystem
  Terminator{,1..3} (4 alike) : Terminator
  World Magnetic Model 2015 : aerolibgravity2/World Magnetic Model 2015  Commented=on  units=Metric (MKS)  time_in=on  month=January  day=1  year=2015  action=Error  h_out=on  dec_out=on  inc_out=on  ti_out=on
      settings: SourceProductName=Aerospace Blockset  SourceProductBaseCode=AE
  B_N : Outport
  V_sun_N : Outport  Port=2
  wires:
  Demux/3 -> World Magnetic Model 2015/1
  Demux/1 -> World Magnetic Model 2015/2
  Demux/2 -> World Magnetic Model 2015/3
  World Magnetic Model 2015/1 -> B_N/1
  World Magnetic Model 2015/2 -> Terminator/1
  World Magnetic Model 2015/3 -> Terminator1/1
  World Magnetic Model 2015/4 -> Terminator2/1
  World Magnetic Model 2015/5 -> Terminator3/1
  x_pos/1 -> ECI Position to LLA/1
  ECI Position to LLA/1 -> Demux/1
  "RBF!!!!! "/1 -> World Magnetic Model 2015/4
  time/1 -> GPS time to Jd sfrom J2000/1(In1), ECI Position to LLA/2
  Normalization/1 -> V_sun_N/1  "s_hat_N"
  GPS time to Jd sfrom J2000/1(Out1) -> Sun position off of Jd frm J2000/1(In1)
  Sun position off of Jd frm J2000/1(Out1) -> Normalization/1

== system Main1/NEW/Flight Computers1/CenterCube EKF/x_measured/q_N from Sensors ==
  B_B : Inport
  V_sun_B : Inport  Port=2
  B_N : Inport  Port=3
  V_sun_N : Inport  Port=4
  Cross Product{1..4} (4 alike) : vrlib/Utilities/Cross Product
      settings: SourceProductBaseCode=VR
  Direction Cosine Matrix to Quaternions : sharedtransform/Direction Cosine Matrix  to Quaternions
      settings: SourceProductName=Aerospace Blockset  SourceProductBaseCode=AE
  Normalization{1..4} (4 alike) : dspmathops/Normalization  NormType=2-norm  Bias=1e-10  NormOver=Each column  Dimension=1  outputDataTypeStr=Inherit: Same as product output  outputLastDataTypeStr=Inherit: Same as product output  outputMin=[]  outputMax=[]  accumDataTypeStr=Inherit: Same as product output  accumLastDataTypeStr=Inherit: Same as product output  roundingMode=Floor  overflowMode=off
      settings: SourceProductName=DSP System Toolbox
  Product : Product  Multiplication=Matrix(*)
  Pseudoinverse : dspinverses/Pseudoinverse  wanterr=off  SimulateUsing=Interpreted execution
      settings: SourceProductName=DSP System Toolbox  SourceProductBaseCode=DS
  Vector Concatenate : Concatenate  NumInputs=3  Mode=Multidimensional array  ConcatenateDimension=2
  Vector Concatenate1 : Concatenate  NumInputs=3  Mode=Multidimensional array  ConcatenateDimension=2
  quat From DCM : Subsystem  Commented=on  TreatAsAtomicUnit=on
  q_N : Outport
  Q : Outport  Port=2
  wires:
  Direction Cosine Matrix to Quaternions/1 -> q_N/1
  V_sun_N/1 -> Cross Product2/1
  V_sun_B/1 -> Cross Product1/1
  B_B/1 -> Cross Product1/2, Normalization2/1
  Cross Product1/1 -> Normalization1/1
  Normalization2/1 -> Vector Concatenate1/2, Cross Product3/1  "b_2"
  Normalization1/1 -> Vector Concatenate1/3, Cross Product3/2  "b_3"
  Cross Product3/1 -> Vector Concatenate1/1  "b_1"
  B_N/1 -> Cross Product2/2, Normalization4/1
  Cross Product2/1 -> Normalization3/1
  Normalization4/1 -> Vector Concatenate/2, Cross Product4/1  "n_2"
  Normalization3/1 -> Vector Concatenate/3, Cross Product4/2  "n_3"
  Cross Product4/1 -> Vector Concatenate/1  "n_1"
  Vector Concatenate/1 -> Product/1
  Product/1 -> Direction Cosine Matrix to Quaternions/1, Q/1
  Pseudoinverse/1 -> Product/2
  Vector Concatenate1/1 -> Pseudoinverse/1

== system Main1/NEW/Sensors1/Center Cube Sensors/Create Sun Vector/GPS time to Jd sfrom J2000 ==
  In1 : Inport
  Jd since GPS0 : Constant  Value=2444244.5
  Jd since J2000 : Constant  Value=2451545
  "Leap Seconds from GSP0 " : Constant  Value=27-9
  Sum : Sum  Inputs=|++
  Sum1 : Sum  Inputs=|++
  Sum2 : Sum  Inputs=|+-
  seconds to days conversion : Gain  Gain=1/86400
  Out1 : Outport
  wires:
  In1/1 -> Sum/1
  "Leap Seconds from GSP0 "/1 -> Sum/2
  Sum/1 -> seconds to days conversion/1
  seconds to days conversion/1 -> Sum1/1
  Jd since GPS0/1 -> Sum1/2
  Sum1/1 -> Sum2/1
  Jd since J2000/1 -> Sum2/2
  Sum2/1 -> Out1/1

== system Main1/NEW/Sensors1/Center Cube Sensors/Create Sun Vector/Sun position off of Jd frm J2000 ==
  In1 : Inport
  Gain : Gain  Gain=1.49597871e8
  MATLAB Function : Subsystem  TreatAsAtomicUnit=on
  Out1 : Outport
  wires:
  In1/1 -> MATLAB Function/1(J2000_days)
  MATLAB Function/1(S_ECI) -> Gain/1
  Gain/1 -> Out1/1

== system Main1/NEW/Sensors1/Center Cube Sensors/Gyro/Bias ==
  w : Inport
  noise : Inport  Port=2
  " Demux " : Demux  Outputs=1
  " SFunction " : S-Function  Tag=Stateflow S-Function Main 22  FunctionName=sf_sfun  PortCounts=[2 2]  SFunctionDeploymentMode=off  EnableBusSupport=on
  " Terminator " : Terminator
  wn : Outport
  wires:
  w/1 -> " SFunction "/1
  noise/1 -> " SFunction "/2
  " SFunction "/2 -> wn/1  "wn"
  " Demux "/1 -> " Terminator "/1
  " SFunction "/1 -> " Demux "/1

== system Main1/NEW/Sensors1/Center Cube Sensors/Magnetometer/Magnetic Field Model ==
  note: IGRF Model
      | Author: Carlos Roithmayr
  r_E : Inport  PortDimensions=[1 3]
  G : Constant  Value=G_igrf
  H : Constant  Value=H_igrf
  IGRF : lib_violet_env/IGRF Model/IGRF
  Kschmidt : Constant  Value=Kschmidt
  R_mean : Constant  Value=R_mean
  b_E : Outport  PortDimensions=3
  wires:
  IGRF/1 -> b_E/1
  R_mean/1 -> IGRF/5
  H/1 -> IGRF/3
  r_E/1 -> IGRF/1
  Kschmidt/1 -> IGRF/4
  G/1 -> IGRF/2

== system Main1/NEW/Flight Computers1/Center Cube Controller/Attitude Compensator/Chart/TorqueD ==
  note: Derivative Controller
      | This controller is a pure derivative controller. It calculates torque to purely oppose the angular velocity. It is better behaved in the short-run than a PD controller projected onto the B field normal plane, but it does not allow for a quaternion command, only a detumble to an unknown attitude.
  note: Regulator
      | - q_target = <input>
      | - w_target = [0 0 0]
  note: Markley Regulator
      | This regulator takes the current directional quaterion vector, the target quaterion, the intertial matrix, and the current angular velocity to determine the required torque necessary to the slew.
      |
      | The equation is 7.8 listed on page 290 of Fundamentals of Spacecraft Attitude Determination and Control. The input I is currently not defined. Also important to the equation is equation 7.2
  w_BN_N : Inport
  I_B : Inport  Port=2
  q : Inport  Port=3
  f : TriggerPort  TriggerType=function-call  VariantControl=(inherit)
      settings: CopyFcn=Stateflow.SLINSF.SimulinkMan.removeBlockPreDeleteFcn  PreDeleteFcn=Stateflow.SLINSF.SimulinkMan.unsafePredeleteFcn
  Display : Display
  Display3 : Display
  Gain3 : Gain  Gain=kd_UD_detumble
  Gain5 : Gain  Gain=-1
  Gain6 : Gain  Commented=on  Gain=1/I_B(1,1)
  Math Function : Math  Operator=transpose  SaturateOnIntegerOverflow=on
  Product2 : Product  Multiplication=Matrix(*)
  Product3 : Product  Inputs=3  Multiplication=Matrix(*)
  Q_B_N : Display
  Quaternions to Direction Cosine Matrix : sharedtransform/Quaternions to  Direction Cosine Matrix
      settings: SourceProductName=Aerospace Blockset  SourceProductBaseCode=AE
  Scope : Scope
  T_N : Outport
  wires:
  Gain3/1 -> T_N/1  "torque_N"
  Product2/1 -> Gain5/1
  Gain5/1 -> Gain3/1
  Product3/1 -> Product2/1, Display/1  "I_N"
  w_BN_N/1 -> Product2/2  "w_BN_N"
  I_B/1 -> Product3/2, Display3/1
  Quaternions to Direction Cosine Matrix/1 -> Q_B_N/1, Product3/3, Math Function/1
  q/1 -> Quaternions to Direction Cosine Matrix/1, Scope/1
  Math Function/1 -> Product3/1

== system Main1/NEW/Flight Computers1/Center Cube Controller/Attitude Compensator/Chart/TorqueDeployed ==
  note: Regulator
      | - q_target = [0 0 0 1]
      | - w_target = [0 0 0]
  q : Inport
  w_BN_N : Inport  Port=2
  f : TriggerPort  TriggerType=function-call  VariantControl=(inherit)
      settings: CopyFcn=Stateflow.SLINSF.SimulinkMan.removeBlockPreDeleteFcn  PreDeleteFcn=Stateflow.SLINSF.SimulinkMan.unsafePredeleteFcn
  Add : Sum
  Gain : Gain  Gain=-1
  Gain1 : Gain  Gain=kp
  Gain2 : Gain  Gain=-1
  Gain3 : Gain  Gain=kd
  Quaternion Inverse : aerolibutil/Quaternion Inverse
      settings: SourceProductName=Aerospace Blockset
  Quaternion Multiplication : aerolibutil/Quaternion Multiplication
  Selector : Selector  InputPortWidth=4  IndexOptions=Index vector (dialog)  Indices=[1 2 3]  OutputSizes=1
  Target q : Constant  Value=[ 0 0 0 1 ]
  T_N : Outport
  wires:
  Gain3/1 -> Gain2/1
  q/1 -> Quaternion Multiplication/1
  Selector/1 -> Gain1/1
  Gain1/1 -> Gain/1
  Quaternion Inverse/1 -> Quaternion Multiplication/2
  Gain2/1 -> Add/2
  Quaternion Multiplication/1 -> Selector/1
  Target q/1 -> Quaternion Inverse/1
  w_BN_N/1 -> Gain3/1
  Gain/1 -> Add/1
  Add/1 -> T_N/1

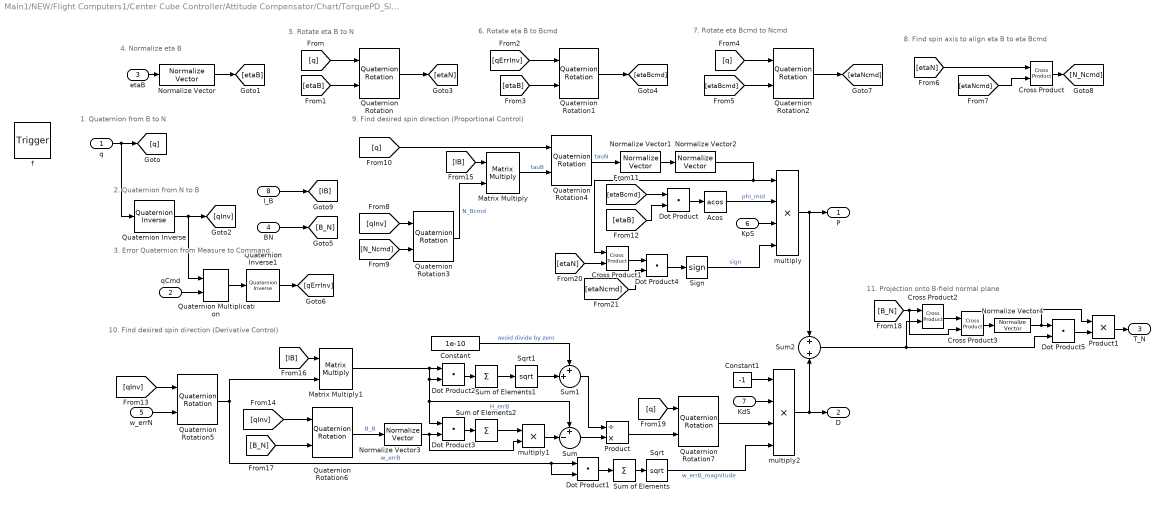
== system Main1/NEW/Flight Computers1/Center Cube Controller/Attitude Compensator/Chart/TorquePD_Slew ==
  note: 1. Quaternion from B to N
  note: 5. Rotate eta B to N
  note: 2. Quaternion from N to B
  note: 3. Error Quaternion from Measure to Command
  note: 6. Rotate eta B to Bcmd
  note: 7. Rotate eta Bcmd to Ncmd
  note: 8. Find spin axis to align eta B to eta Bcmd
  note: 9. Find desired spin direction (Proportional Control)
  note: 10. Find desired spin direction (Derivative Control)
  note: 4. Normalize eta B
  note: 11. Projection onto B-field normal plane
  q : Inport
  qCmd : Inport  Port=2
  etaB : Inport  Port=3
  BN : Inport  Port=4
  w_errN : Inport  Port=5
  KpS : Inport  Port=6
  KdS : Inport  Port=7
  I_B : Inport  Port=8
  f : TriggerPort  TriggerType=function-call  VariantControl=(inherit)
      settings: CopyFcn=Stateflow.SLINSF.SimulinkMan.removeBlockPreDeleteFcn  PreDeleteFcn=Stateflow.SLINSF.SimulinkMan.unsafePredeleteFcn
  Acos : Trigonometry  Operator=acos
  Constant : Constant  Value=1e-10
  Constant1 : Constant  Value=-1
  Cross Product{,1..3} (4 alike) : vrlib/Utilities/Cross Product
      settings: SourceProductBaseCode=VR
  Dot Product{,1..5} (6 alike) : DotProduct  InputSameDT=on  OutDataTypeStr=Inherit: Inherit via internal rule
  Matrix Multiply : Product  Multiplication=Matrix(*)
  Matrix Multiply1 : Product  Multiplication=Matrix(*)
  Normalize Vector{,1..4} (5 alike) : vrlib/Utilities/Normalize Vector  maxzero=0
      settings: SourceProductName=Simulink 3D Animation  SourceProductBaseCode=VR
  Product : Product  Inputs=/*
  Product1 : Product
  Quaternion Inverse : aerolibutil/Quaternion Inverse
      settings: SourceProductName=Aerospace Blockset
  Quaternion Inverse1 : aerolibutil/Quaternion Inverse
      settings: SourceProductName=Aerospace Blockset
  Quaternion Multiplication : aerolibutil/Quaternion Multiplication
  Quaternion Rotation{,1..7} (8 alike) : aerolibutil/Quaternion Rotation
  Sign : Signum
  Sqrt : Sqrt  SaturateOnIntegerOverflow=on
  Sqrt1 : Sqrt  SaturateOnIntegerOverflow=on
  Sum : Sum  Inputs=+-|
  Sum of Elements : Sum  Inputs=+
  Sum of Elements1 : Sum  Inputs=+
  Sum of Elements2 : Sum  Inputs=+
  Sum1 : Sum  Inputs=++|
  Sum2 : Sum
  multiply : Product  Inputs=****
  multiply1 : Product  Inputs=**
  multiply2 : Product  Inputs=****
  P : Outport
  D : Outport  Port=2
  T_N : Outport  Port=3
  wires:
  etaB/1 -> Normalize Vector/1
  Quaternion Rotation/1 -> [etaN]
  q/1 -> [q], Quaternion Inverse/1
  [q] -> Quaternion Rotation/1
  Normalize Vector/1 -> [etaB]
  [etaB] -> Quaternion Rotation/2
  Quaternion Inverse/1 -> Quaternion Multiplication/1, [qInv]
  [qErrInv] -> Quaternion Rotation1/1
  [etaB] -> Quaternion Rotation1/2
  Quaternion Rotation1/1 -> [etaBcmd]
  qCmd/1 -> Quaternion Multiplication/2
  Quaternion Multiplication/1 -> Quaternion Inverse1/1
  Quaternion Inverse1/1 -> [qErrInv]
  [q] -> Quaternion Rotation2/1
  [etaBcmd] -> Quaternion Rotation2/2
  Quaternion Rotation2/1 -> [etaNcmd]
  [etaN] -> Cross Product/1
  [etaNcmd] -> Cross Product/2
  Cross Product/1 -> [N_Ncmd]
  Quaternion Rotation3/1 -> Matrix Multiply/2  "N_Bcmd"
  [N_Ncmd] -> Quaternion Rotation3/2
  [qInv] -> Quaternion Rotation3/1
  [q] -> Quaternion Rotation4/1
  Matrix Multiply/1 -> Quaternion Rotation4/2  "tauB"
  Quaternion Rotation4/1 -> Normalize Vector1/1  "tauN"
  Normalize Vector1/1 -> Normalize Vector2/1
  Normalize Vector2/1 -> Cross Product1/1, multiply/1
  Dot Product/1 -> Acos/1
  [etaB] -> Dot Product/2
  [etaBcmd] -> Dot Product/1
  Acos/1 -> multiply/2  "phi_mid"
  KpS/1 -> multiply/3
  multiply/1 -> P/1, Sum2/1
  [qInv] -> Quaternion Rotation5/1
  w_errN/1 -> Quaternion Rotation5/2
  [qInv] -> Quaternion Rotation6/1
  Quaternion Rotation6/1 -> Normalize Vector3/1  "B_B"
  I_B/1 -> [IB]
  [IB] -> Matrix Multiply/1
  [IB] -> Matrix Multiply1/1
  Quaternion Rotation5/1 -> Dot Product1/1, Dot Product1/2, Matrix Multiply1/2  "w_errB"
  Normalize Vector3/1 -> Dot Product3/2, multiply1/2
  Constant/1 -> Sum1/1  "avoid divide by zero"
  [q] -> Quaternion Rotation7/1
  Sum/1 -> Product/2
  Sum1/1 -> Product/1
  Product/1 -> Quaternion Rotation7/2
  Sqrt1/1 -> Sum1/2
  Matrix Multiply1/1 -> Sum/1, Dot Product3/1, Dot Product2/2, Dot Product2/1  "H_errB"
  Dot Product1/1 -> Sum of Elements/1
  Sum of Elements/1 -> Sqrt/1
  Sum of Elements1/1 -> Sqrt1/1
  Dot Product2/1 -> Sum of Elements1/1
  [etaN] -> Cross Product1/2
  Cross Product1/1 -> Dot Product4/1
  [etaNcmd] -> Dot Product4/2
  Dot Product4/1 -> Sign/1
  Sign/1 -> multiply/4  "sign"
  multiply1/1 -> Sum/2
  Dot Product3/1 -> Sum of Elements2/1
  Sum of Elements2/1 -> multiply1/1
  Quaternion Rotation7/1 -> multiply2/3
  KdS/1 -> multiply2/2
  Constant1/1 -> multiply2/1
  multiply2/1 -> D/1, Sum2/2
  Sqrt/1 -> multiply2/4  "w_errB_magnitude"
  Normalize Vector4/1 -> Product1/1, Dot Product5/1
  Cross Product2/1 -> Cross Product3/1
  [B_N] -> Cross Product2/1, Cross Product3/2
  Cross Product3/1 -> Normalize Vector4/1
  Sum2/1 -> Cross Product2/2, Dot Product5/2
  Product1/1 -> T_N/1
  Dot Product5/1 -> Product1/2
  BN/1 -> [B_N]
  [B_N] -> Quaternion Rotation6/2
